simulink model "spindle_sensoryneuron"  (Simulink 7.8)
settings: Solver=ode2  StartTime=0.0  StopTime=4  FixedStep=T  RelTol=1e-3
InitFcn:
  | [A tau T] = emg_filter();
  | up = generate_min_jerk( 1, 1.1, 2.0, T );
  | down = 2.1 - up;
  | stretch = [repmat([up; down], 2, 1); [up ;down]];
  | l = length(stretch);
  | stretch(1 : ceil(l/3), 2) = 1;
  | stretch(:, 1) = [0:l-1]*T;
  | 
  | mag1 = 48144;
  | mag2 = 45845;
  | trise = 0.02;
  | tfall  = 0.04;
  | [num_syn den_syn] = filter_coef(mag1, mag2, trise, tfall,T)
  | 
  | for i = 1:20
  |     eval(['SIZE_MU_', num2str(i), '=', num2str('(atan(150) - atan(i^0.8)) * 6;')])
  | end
StopFcn:
  | %recruitment_pattern_plotter(spikes_g1, spikes_g2, total_force, 0.02)
  | %incrementVars('emg_spasticity')
undefined symbols (not defined in the file or in its folder): SIZE_MU_1, SIZE_MU_10, SIZE_MU_2, SIZE_MU_3, SIZE_MU_4, SIZE_MU_5, SIZE_MU_6, SIZE_MU_7, SIZE_MU_8, SIZE_MU_9, T
libraries: simulink x9
settings Model: Creator=minos_niu  LastModifiedBy=minos_niu

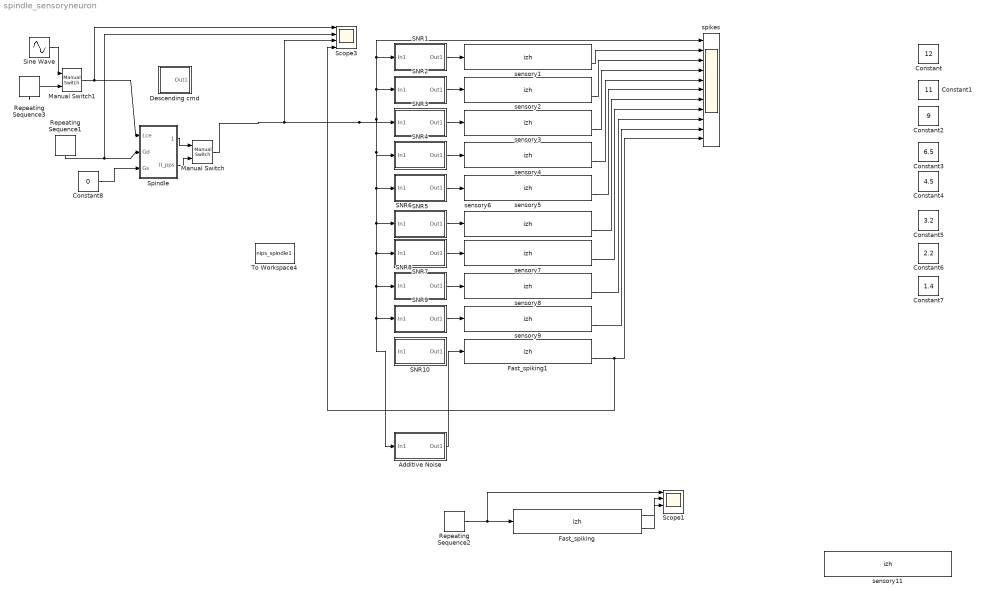
== system spindle_sensoryneuron ==
  Additive Noise : Subsystem
  Constant : Constant  Value=12
  Constant1 : Constant  Value=11
  Constant2 : Constant  Value=9
  Constant3 : Constant  Value=6.5
  Constant4 : Constant  Value=4.5
  Constant5 : Constant  Value=3.2
  Constant6 : Constant  Value=2.2
  Constant7 : Constant  Value=1.4
  Constant8 : Constant  Value=0
  Descending cmd : Subsystem
  Fast_spiking : S-Function  FunctionName=izh  Parameters=[0.01 0.2 -65.0 2.0 30.0 SIZE_MU_10] [-70.0 -14.0]  EnableBusSupport=off
      mask Display:
      | port_label('input', 1, 'syn curr');
      | port_label('output', 1, 'action potential');
      | port_label('output', 2, 'spike');
      | disp('Izhi Neuron \n(S-Function)')
  Fast_spiking1 : S-Function  FunctionName=izh  Parameters=[0.01 0.2 -65.0 2.0 30.0 SIZE_MU_10] [-70.0 -14.0]  EnableBusSupport=off
      mask Display:
      | port_label('input', 1, 'syn curr');
      | port_label('output', 1, 'action potential');
      | port_label('output', 2, 'spike');
      | disp('Izhi Neuron \n(S-Function)')
  Manual Switch : simulink/Signal Routing/Manual Switch  sw=1  action=0  varsize=off
  Manual Switch1 : simulink/Signal Routing/Manual Switch  sw=1  action=0  varsize=off
  Repeating Sequence1 : simulink/Sources/Repeating Sequence  rep_seq_t=[0 1.8 2.1 4.0]  rep_seq_y=[1.00 1.0 80.0 80.0]
  Repeating Sequence2 : simulink/Sources/Repeating Sequence  rep_seq_t=[0 0.3 4.0]  rep_seq_y=[0 0 45 ]
  Repeating Sequence3 : simulink/Sources/Repeating Sequence  rep_seq_t=[0 1.3 1.5 4.0]  rep_seq_y=[1.00 1.0 1.04 1.04]
  SNR1 : Subsystem
  SNR10 : Subsystem
  SNR2 : Subsystem
  SNR3 : Subsystem
  SNR4 : Subsystem
  SNR5 : Subsystem
  SNR6 : Subsystem
  SNR7 : Subsystem
  SNR8 : Subsystem
  SNR9 : Subsystem
  Scope1 : Scope  NumInputPorts=4
      settings: TimeRange=10  YMin=0~-5~-5~-5  YMax=37.5~5~5~5  SaveName=total_force  DataFormat=Structure
  Scope3 : Scope  NumInputPorts=4
      settings: TimeRange=10  YMin=0~-5~-5~-5  YMax=37.5~5~5~5  SaveName=total_force2  DataFormat=Structure
  Sine Wave : Sin  Amplitude=0.1  Bias=1.1  Frequency=2*pi*2  Phase=-pi/2  SampleTime=T
  Spindle : Subsystem
  To Workspace4 : ToWorkspace  VariableName=nips_spindle1  SampleTime=-1  SaveFormat=Structure With Time
  sensory1 : S-Function  FunctionName=izh  Parameters=[0.02 0.2 -65.0 6.0 30.0 SIZE_MU_1] [-70.0 -14.0]  EnableBusSupport=off
      mask Display:
      | port_label('input', 1, 'syn curr');
      | port_label('output', 1, 'action potential');
      | port_label('output', 2, 'spike');
      | disp('Izhi Neuron \n(S-Function)')
  sensory11 : S-Function  FunctionName=izh  Parameters=[0.02 0.2 -65.0 6.0 30.0 SIZE_MU_10] [-70.0 -14.0]  EnableBusSupport=off
      mask Display:
      | port_label('input', 1, 'syn curr');
      | port_label('output', 1, 'action potential');
      | port_label('output', 2, 'spike');
      | disp('Izhi Neuron \n(S-Function)')
  sensory2 : S-Function  FunctionName=izh  Parameters=[0.02 0.2 -65.0 6.0 30.0 SIZE_MU_2] [-70.0 -14.0]  EnableBusSupport=off
      mask Display:
      | port_label('input', 1, 'syn curr');
      | port_label('output', 1, 'action potential');
      | port_label('output', 2, 'spike');
      | disp('Izhi Neuron \n(S-Function)')
  sensory3 : S-Function  FunctionName=izh  Parameters=[0.02 0.2 -65.0 6.0 30.0 SIZE_MU_3] [-70.0 -14.0]  EnableBusSupport=off
      mask Display:
      | port_label('input', 1, 'syn curr');
      | port_label('output', 1, 'action potential');
      | port_label('output', 2, 'spike');
      | disp('Izhi Neuron \n(S-Function)')
  sensory4 : S-Function  FunctionName=izh  Parameters=[0.02 0.2 -65.0 6.0 30.0 SIZE_MU_4] [-70.0 -14.0]  EnableBusSupport=off
      mask Display:
      | port_label('input', 1, 'syn curr');
      | port_label('output', 1, 'action potential');
      | port_label('output', 2, 'spike');
      | disp('Izhi Neuron \n(S-Function)')
  sensory5 : S-Function  FunctionName=izh  Parameters=[0.02 0.2 -65.0 6.0 30.0 SIZE_MU_5] [-70.0 -14.0]  EnableBusSupport=off
      mask Display:
      | port_label('input', 1, 'syn curr');
      | port_label('output', 1, 'action potential');
      | port_label('output', 2, 'spike');
      | disp('Izhi Neuron \n(S-Function)')
  sensory6 : S-Function  FunctionName=izh  Parameters=[0.02 0.2 -65.0 6.0 30.0 SIZE_MU_6] [-70.0 -14.0]  EnableBusSupport=off
      mask Display:
      | port_label('input', 1, 'syn curr');
      | port_label('output', 1, 'action potential');
      | port_label('output', 2, 'spike');
      | disp('Izhi Neuron \n(S-Function)')
  sensory7 : S-Function  FunctionName=izh  Parameters=[0.02 0.2 -65.0 6.0 30.0 SIZE_MU_7] [-70.0 -14.0]  EnableBusSupport=off
      mask Display:
      | port_label('input', 1, 'syn curr');
      | port_label('output', 1, 'action potential');
      | port_label('output', 2, 'spike');
      | disp('Izhi Neuron \n(S-Function)')
  sensory8 : S-Function  FunctionName=izh  Parameters=[0.02 0.2 -65.0 6.0 30.0 SIZE_MU_8] [-70.0 -14.0]  EnableBusSupport=off
      mask Display:
      | port_label('input', 1, 'syn curr');
      | port_label('output', 1, 'action potential');
      | port_label('output', 2, 'spike');
      | disp('Izhi Neuron \n(S-Function)')
  sensory9 : S-Function  FunctionName=izh  Parameters=[0.02 0.2 -65.0 6.0 30.0 SIZE_MU_9] [-70.0 -14.0]  EnableBusSupport=off
      mask Display:
      | port_label('input', 1, 'syn curr');
      | port_label('output', 1, 'action potential');
      | port_label('output', 2, 'spike');
      | disp('Izhi Neuron \n(S-Function)')
  spikes : Scope  NumInputPorts=11
      settings: TickLabels=on  TimeRange=5  YMin=-1000~-5~-5~-5~-5~-5~-5~-5~-5~-5~-5  YMax=5000~5~5~5~5~5~5~5~5~5~5  SaveName=spikes_g1  DataFormat=Structure
  wires:
  sensory1/2 -> spikes/2
  sensory2/2 -> spikes/3
  sensory3/2 -> spikes/4
  sensory4/2 -> spikes/5
  sensory5/2 -> spikes/6
  sensory6/2 -> spikes/7
  sensory7/2 -> spikes/8
  sensory9/2 -> spikes/10
  Fast_spiking1/2 -> spikes/11, Scope3/4
  sensory8/2 -> spikes/9
  SNR1/1(Out1) -> sensory1/1
  SNR2/1(Out1) -> sensory2/1
  SNR3/1(Out1) -> sensory3/1
  SNR4/1(Out1) -> sensory4/1
  SNR5/1(Out1) -> sensory5/1
  SNR6/1(Out1) -> sensory6/1
  SNR7/1(Out1) -> sensory7/1
  SNR8/1(Out1) -> sensory8/1
  SNR9/1(Out1) -> sensory9/1
  Constant8/1 -> Spindle/3(Gs)
  Spindle/1(Ia_pps) -> Manual Switch/1
  Spindle/2(II_pps) -> Manual Switch/2
  Manual Switch/1 -> SNR2/1(In1), SNR1/1(In1), spikes/1, SNR4/1(In1), SNR5/1(In1), SNR6/1(In1), SNR7/1(In1), SNR8/1(In1), SNR9/1(In1), Additive Noise/1(In1), SNR3/1(In1), Scope3/3
  Repeating Sequence2/1 -> Fast_spiking/1, Scope1/1
  Fast_spiking/1 -> Scope1/2
  Fast_spiking/2 -> Scope1/3
  Additive Noise/1(Out1) -> Fast_spiking1/1
  Manual Switch1/1 -> Spindle/1(Lce), Scope3/1
  Sine Wave/1 -> Manual Switch1/1
  Repeating Sequence3/1 -> Manual Switch1/2
  Repeating Sequence1/1 -> Spindle/2(Gd), Scope3/2

== system spindle_sensoryneuron/Additive Noise ==
  In1 : Inport
  Add : Sum
  Scope : Scope
  Uniform Random Number : UniformRandomNumber  Minimum=-1.0  Maximum=1.0  SampleTime=T
  Out1 : Outport
  wires:
  Add/1 -> Scope/1, Out1/1
  In1/1 -> Add/1
  Uniform Random Number/1 -> Add/2

== system spindle_sensoryneuron/Descending cmd ==
  Add2 : Sum
  Descending1 : simulink/Sources/Repeating Sequence  rep_seq_t=[0 1.1 3.1 6.8 9.5 10 ]  rep_seq_y=[0 0 20 20 0 0]*1
  Descending2 : simulink/Sources/Repeating Sequence  rep_seq_t=[0 0.5 1]  rep_seq_y=[0 200 200]*0
  Manual Switch : simulink/Signal Routing/Manual Switch  sw=0  action=0  varsize=off
  Uniform Random Number : UniformRandomNumber  Minimum=-6  Maximum=0  SampleTime=T
  Out1 : Outport
  wires:
  Manual Switch/1 -> Out1/1
  Add2/1 -> Manual Switch/1
  Uniform Random Number/1 -> Add2/2
  Descending2/1 -> Manual Switch/2
  Descending1/1 -> Add2/1

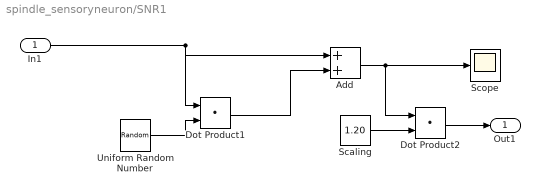
== system spindle_sensoryneuron/SNR1 ==
  In1 : Inport
  Add : Sum
  Dot Product1 : DotProduct  InputSameDT=on  OutDataTypeStr=Inherit: Inherit via internal rule
  Dot Product2 : DotProduct  InputSameDT=on  OutDataTypeStr=Inherit: Inherit via internal rule
  Scaling : Constant  Value=1.20  SampleTime=T
  Scope : Scope
  Uniform Random Number : UniformRandomNumber  Minimum=-0.3  Maximum=0.3  SampleTime=T
  Out1 : Outport
  wires:
  Scaling/1 -> Dot Product2/2
  Dot Product2/1 -> Out1/1
  Add/1 -> Dot Product2/1, Scope/1
  Dot Product1/1 -> Add/2
  In1/1 -> Add/1, Dot Product1/1
  Uniform Random Number/1 -> Dot Product1/2

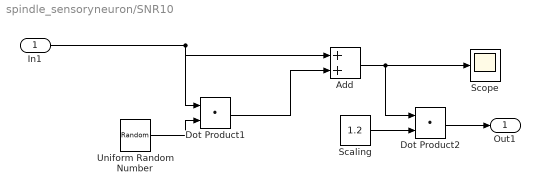
== system spindle_sensoryneuron/SNR10 ==
  In1 : Inport
  Add : Sum
  Dot Product1 : DotProduct  InputSameDT=on  OutDataTypeStr=Inherit: Inherit via internal rule
  Dot Product2 : DotProduct  InputSameDT=on  OutDataTypeStr=Inherit: Inherit via internal rule
  Scaling : Constant  Value=1.2
  Scope : Scope
  Uniform Random Number : UniformRandomNumber  Minimum=-0.3  Maximum=0.3  SampleTime=T
  Out1 : Outport
  wires:
  Scaling/1 -> Dot Product2/2
  Dot Product2/1 -> Out1/1
  Add/1 -> Dot Product2/1, Scope/1
  Dot Product1/1 -> Add/2
  In1/1 -> Add/1, Dot Product1/1
  Uniform Random Number/1 -> Dot Product1/2

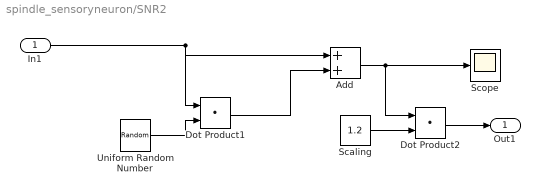
== system spindle_sensoryneuron/SNR2 ==
  In1 : Inport
  Add : Sum
  Dot Product1 : DotProduct  InputSameDT=on  OutDataTypeStr=Inherit: Inherit via internal rule
  Dot Product2 : DotProduct  InputSameDT=on  OutDataTypeStr=Inherit: Inherit via internal rule
  Scaling : Constant  Value=1.2
  Scope : Scope
  Uniform Random Number : UniformRandomNumber  Minimum=-0.3  Maximum=0.3  SampleTime=T
  Out1 : Outport
  wires:
  Scaling/1 -> Dot Product2/2
  Dot Product2/1 -> Out1/1
  Add/1 -> Dot Product2/1, Scope/1
  Dot Product1/1 -> Add/2
  In1/1 -> Add/1, Dot Product1/1
  Uniform Random Number/1 -> Dot Product1/2

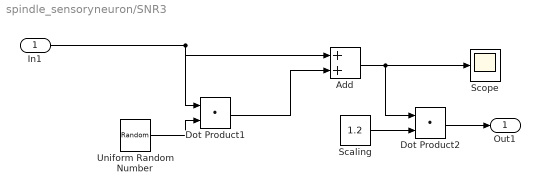
== system spindle_sensoryneuron/SNR3 ==
  In1 : Inport
  Add : Sum
  Dot Product1 : DotProduct  InputSameDT=on  OutDataTypeStr=Inherit: Inherit via internal rule
  Dot Product2 : DotProduct  InputSameDT=on  OutDataTypeStr=Inherit: Inherit via internal rule
  Scaling : Constant  Value=1.2
  Scope : Scope
  Uniform Random Number : UniformRandomNumber  Minimum=-0.3  Maximum=0.3  SampleTime=T
  Out1 : Outport
  wires:
  Scaling/1 -> Dot Product2/2
  Dot Product2/1 -> Out1/1
  Add/1 -> Dot Product2/1, Scope/1
  Dot Product1/1 -> Add/2
  In1/1 -> Add/1, Dot Product1/1
  Uniform Random Number/1 -> Dot Product1/2

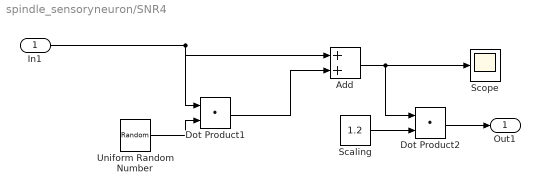
== system spindle_sensoryneuron/SNR4 ==
  In1 : Inport
  Add : Sum
  Dot Product1 : DotProduct  InputSameDT=on  OutDataTypeStr=Inherit: Inherit via internal rule
  Dot Product2 : DotProduct  InputSameDT=on  OutDataTypeStr=Inherit: Inherit via internal rule
  Scaling : Constant  Value=1.2
  Scope : Scope
  Uniform Random Number : UniformRandomNumber  Minimum=-0.3  Maximum=0.3  SampleTime=T
  Out1 : Outport
  wires:
  Scaling/1 -> Dot Product2/2
  Dot Product2/1 -> Out1/1
  Add/1 -> Dot Product2/1, Scope/1
  Dot Product1/1 -> Add/2
  In1/1 -> Add/1, Dot Product1/1
  Uniform Random Number/1 -> Dot Product1/2

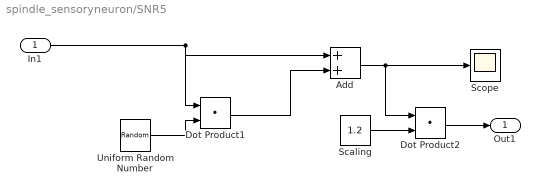
== system spindle_sensoryneuron/SNR5 ==
  In1 : Inport
  Add : Sum
  Dot Product1 : DotProduct  InputSameDT=on  OutDataTypeStr=Inherit: Inherit via internal rule
  Dot Product2 : DotProduct  InputSameDT=on  OutDataTypeStr=Inherit: Inherit via internal rule
  Scaling : Constant  Value=1.2
  Scope : Scope
  Uniform Random Number : UniformRandomNumber  Minimum=-0.3  Maximum=0.3  SampleTime=T
  Out1 : Outport
  wires:
  Scaling/1 -> Dot Product2/2
  Dot Product2/1 -> Out1/1
  Add/1 -> Dot Product2/1, Scope/1
  Dot Product1/1 -> Add/2
  In1/1 -> Add/1, Dot Product1/1
  Uniform Random Number/1 -> Dot Product1/2

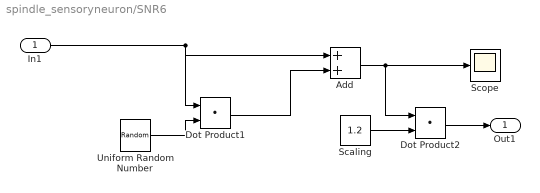
== system spindle_sensoryneuron/SNR6 ==
  In1 : Inport
  Add : Sum
  Dot Product1 : DotProduct  InputSameDT=on  OutDataTypeStr=Inherit: Inherit via internal rule
  Dot Product2 : DotProduct  InputSameDT=on  OutDataTypeStr=Inherit: Inherit via internal rule
  Scaling : Constant  Value=1.2
  Scope : Scope
  Uniform Random Number : UniformRandomNumber  Minimum=-0.3  Maximum=0.3  SampleTime=T
  Out1 : Outport
  wires:
  Scaling/1 -> Dot Product2/2
  Dot Product2/1 -> Out1/1
  Add/1 -> Dot Product2/1, Scope/1
  Dot Product1/1 -> Add/2
  In1/1 -> Add/1, Dot Product1/1
  Uniform Random Number/1 -> Dot Product1/2

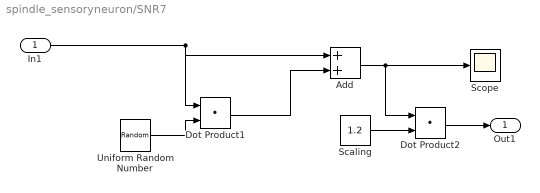
== system spindle_sensoryneuron/SNR7 ==
  In1 : Inport
  Add : Sum
  Dot Product1 : DotProduct  InputSameDT=on  OutDataTypeStr=Inherit: Inherit via internal rule
  Dot Product2 : DotProduct  InputSameDT=on  OutDataTypeStr=Inherit: Inherit via internal rule
  Scaling : Constant  Value=1.2
  Scope : Scope
  Uniform Random Number : UniformRandomNumber  Minimum=-0.3  Maximum=0.3  SampleTime=T
  Out1 : Outport
  wires:
  Scaling/1 -> Dot Product2/2
  Dot Product2/1 -> Out1/1
  Add/1 -> Dot Product2/1, Scope/1
  Dot Product1/1 -> Add/2
  In1/1 -> Add/1, Dot Product1/1
  Uniform Random Number/1 -> Dot Product1/2

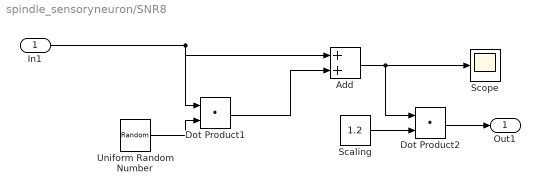
== system spindle_sensoryneuron/SNR8 ==
  In1 : Inport
  Add : Sum
  Dot Product1 : DotProduct  InputSameDT=on  OutDataTypeStr=Inherit: Inherit via internal rule
  Dot Product2 : DotProduct  InputSameDT=on  OutDataTypeStr=Inherit: Inherit via internal rule
  Scaling : Constant  Value=1.2
  Scope : Scope
  Uniform Random Number : UniformRandomNumber  Minimum=-0.3  Maximum=0.3  SampleTime=T
  Out1 : Outport
  wires:
  Scaling/1 -> Dot Product2/2
  Dot Product2/1 -> Out1/1
  Add/1 -> Dot Product2/1, Scope/1
  Dot Product1/1 -> Add/2
  In1/1 -> Add/1, Dot Product1/1
  Uniform Random Number/1 -> Dot Product1/2

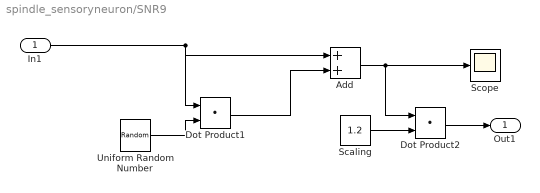
== system spindle_sensoryneuron/SNR9 ==
  In1 : Inport
  Add : Sum
  Dot Product1 : DotProduct  InputSameDT=on  OutDataTypeStr=Inherit: Inherit via internal rule
  Dot Product2 : DotProduct  InputSameDT=on  OutDataTypeStr=Inherit: Inherit via internal rule
  Scaling : Constant  Value=1.2
  Scope : Scope
  Uniform Random Number : UniformRandomNumber  Minimum=-0.3  Maximum=0.3  SampleTime=T
  Out1 : Outport
  wires:
  Scaling/1 -> Dot Product2/2
  Dot Product2/1 -> Out1/1
  Add/1 -> Dot Product2/1, Scope/1
  Dot Product1/1 -> Add/2
  In1/1 -> Add/1, Dot Product1/1
  Uniform Random Number/1 -> Dot Product1/2

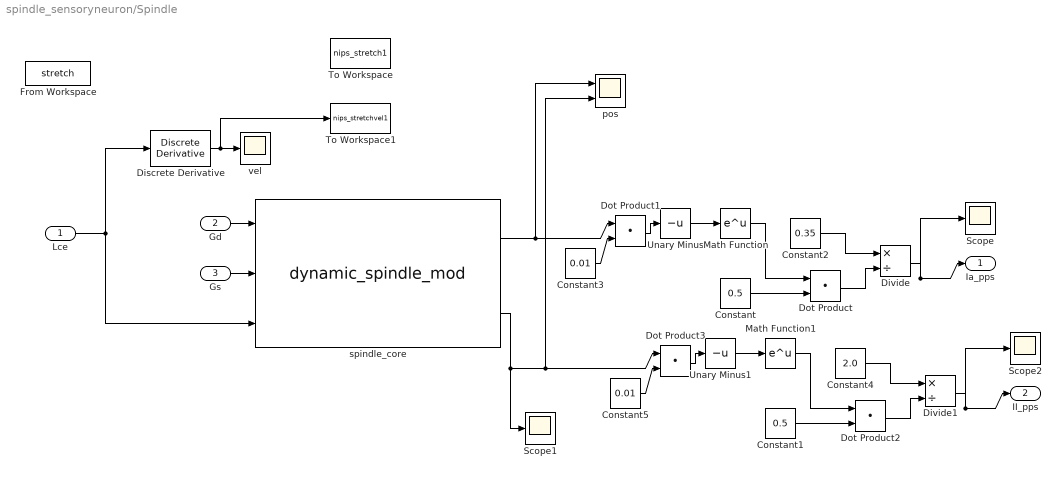
== system spindle_sensoryneuron/Spindle ==
  Lce : Inport
  Gd : Inport  Port=2
  Gs : Inport  Port=3
  Constant : Constant  Value=0.5
  Constant1 : Constant  Value=0.5
  Constant2 : Constant  Value=0.35
  Constant3 : Constant  Value=0.01
  Constant4 : Constant  Value=2.0
  Constant5 : Constant  Value=0.01
  Discrete Derivative : simulink/Discrete/Discrete Derivative  gainval=1.0  ICPrevScaledInput=0  InputProcessing=Inherited  OutMin=[]  OutMax=[]  OutDataType=fixdt(1, 16)  OutScaling=2^-10  DoSatur=off
  Divide : Product  Inputs=*/
  Divide1 : Product  Inputs=*/
  Dot Product{,1..3} (4 alike) : DotProduct  InputSameDT=on  OutDataTypeStr=Inherit: Inherit via internal rule
  From Workspace : FromWorkspace  VariableName=stretch  SampleTime=T
  Math Function : Math  SaturateOnIntegerOverflow=on
  Math Function1 : Math  SaturateOnIntegerOverflow=on
  Scope : Scope
      settings: YMin=0  YMax=225
  Scope1 : Scope
      settings: TimeRange=1  SaveName=ScopeData4
  Scope2 : Scope
      settings: YMin=0  YMax=225  SaveName=ScopeData2
  To Workspace : ToWorkspace  VariableName=nips_stretch1  SampleTime=-1  SaveFormat=Structure With Time
  To Workspace1 : ToWorkspace  VariableName=nips_stretchvel1  SampleTime=-1  SaveFormat=Structure With Time
  Unary Minus : UnaryMinus
  Unary Minus1 : UnaryMinus
  pos : Scope  NumInputPorts=2
      settings: YMin=-5~-5  YMax=5~5  SaveName=ScopeData5
  spindle_core : S-Function  FunctionName=dynamic_spindle_mod  Parameters=[10.4649 10.4649 10.4649] [0.1127 0.1623 0.1623] [0.0605 0.0822 0.0822] [0.2356 -0.046 -0.069] [0 0 0] [0.0289 0.0636 0.0954] [1 0.7 0.7] [1 0.92 0.92] [20000 10000 10000] [20000 7250 7250] [0.3 0.3 0.3] [0.46 0.46 0.46] [0.04 0.04 0.04] [0.76 0.76 0.76] [1 0.04 0.04] [0.192 0.185 0.0001] [0.0002 0.0002 0.0002] [1 0.5 1] [1]  EnableBusSupport=off
      mask Display:
      | port_label('input', 1, 'gamma dynamic');
      | port_label('input', 2, 'gamma static');
      | port_label('input', 3, 'Lce(L0)');
      | port_label('output',1,'Ia');
      | port_label('output',2,'II');
      | disp('Muscle Spindle \n(S-Function)')
  vel : Scope
      settings: SaveName=ScopeData6
  Ia_pps : Outport
  II_pps : Outport  Port=2
  wires:
  Discrete Derivative/1 -> vel/1, To Workspace1/1
  spindle_core/1 -> Dot Product1/1, pos/1
  spindle_core/2 -> Scope1/1, Dot Product3/1, pos/2
  Math Function/1 -> Dot Product/1
  Constant/1 -> Dot Product/2
  Unary Minus/1 -> Math Function/1
  Constant2/1 -> Divide/1
  Dot Product/1 -> Divide/2
  Divide/1 -> Ia_pps/1, Scope/1
  Constant3/1 -> Dot Product1/2
  Dot Product1/1 -> Unary Minus/1
  Lce/1 -> Discrete Derivative/1, spindle_core/3
  Gd/1 -> spindle_core/1
  Gs/1 -> spindle_core/2
  Math Function1/1 -> Dot Product2/1
  Constant1/1 -> Dot Product2/2
  Unary Minus1/1 -> Math Function1/1
  Constant4/1 -> Divide1/1
  Dot Product2/1 -> Divide1/2
  Divide1/1 -> II_pps/1, Scope2/1
  Constant5/1 -> Dot Product3/2
  Dot Product3/1 -> Unary Minus1/1
